simulink model "Filter_Sim_8th_Order"  (R2017a)
settings: Solver=VariableStepAuto  StartTime=0.0  StopTime=t_stop  RelTol=1e-3
values from neighbouring files (symbols this model uses):
  alpha = den_ts    [Filter_Sim.m]
  b_frac = qs    [Filter_Sim.m]
  beta = num_ts    [Filter_Sim.m]
  bw = bi + qs + 1    [Filter_Sim.m]
  bw_accum = 1 + ceil(abs(log2(ts))) + b_frac(2:end)    [Filter_Sim.m]
  k = zeros(1,length(f_norm))    [dIIR_scaling.m]
  shift = round(abs(log2(ts*k)))    [Filter_Sim.m]
  ts = 1/fs    (= 8.85770975057e-08)    [Filter_Sim.m]
libraries: xbsIndex_r4 x117
settings Model: Creator=jpoverelli  LastModifiedBy=jpoverelli

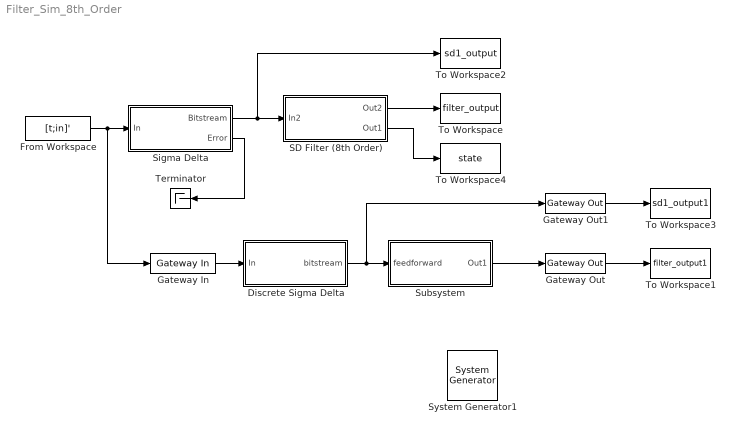
== system Filter_Sim_8th_Order ==
  " System Generator1" : xbsIndex_r4/ System Generator  Tag=genX  xilinxfamily=spartan7  part=xc7s50  speed=-2  package=ftgb196  synthesis_tool=Vivado  clock_wrapper=Clock Enables  directory=/home/jpoverelli/Desktop/Sigma_Delta_Filter_Design/Matlab_Files/Filter_Design/netlist  proj_type=Vivado  Synth_file=Vivado Synthesis Defaults  Impl_file=Vivado Implementation Defaults  testbench=off  simulink_period=ts  sysclk_period=ts/1e-9  dcm_input_clock_period=10  incr_netlist=off  trim_vbits=Everywhere in SubSystem  dbl_ovrd=According to Block Masks  core_generation=According to Block Masks  run_coregen=off  deprecated_control=off  eval_field=0  block_type=sysgen
  Discrete Sigma Delta : Subsystem  mask{bw=bw(1), frac=b_frac(1)}
  From Workspace : FromWorkspace  VariableName=[t;in]'  SampleTime=ts
  Gateway In : xbsIndex_r4/Gateway In  gui_display_data_type=Fixed-point  arith_type="Signed  (2's comp)"  n_bits=bw(1)  bin_pt=b_frac(1)  preci_type=Single  exp_width=8  frac_width=24  rows=1  columns=1  quantization="Round  (unbiased: +/- Inf)"  overflow=Saturate  period=ts  UseAsADC=off  ADCChannel='1'  interface=None  automatic_assignment=on  address_offset=hex2dec('00')  intf_name=''  intf_description=''  default_value=0  timing_constraint=None  locs_specified=off  LOCs={}  io_standard={}  inherit_from_input=off  hdl_port=on  dbl_ovrd=off  block_type=gatewayin
  Gateway Out : xbsIndex_r4/Gateway Out  inherit_from_input=off  hdl_port=on  rows=1  columns=1  UseAsDAC=off  DACChannel='1'  interface=None  automatic_assignment=on  address_offset=hex2dec('00')  intf_name=''  intf_description=''  timing_constraint=None  locs_specified=off  LOCs={}  io_standard={}  block_type=gatewayout
  Gateway Out1 : xbsIndex_r4/Gateway Out  inherit_from_input=off  hdl_port=on  rows=1  columns=1  UseAsDAC=off  DACChannel='1'  interface=None  automatic_assignment=on  address_offset=hex2dec('00')  intf_name=''  intf_description=''  timing_constraint=None  locs_specified=off  LOCs={}  io_standard={}  block_type=gatewayout
  SD Filter (8th Order) : Subsystem
  Sigma Delta : Subsystem
  Subsystem : Subsystem
  Terminator : Terminator
  To Workspace : ToWorkspace  VariableName=filter_output  SampleTime=-1
  To Workspace1 : ToWorkspace  VariableName=filter_output1  SampleTime=-1
  To Workspace2 : ToWorkspace  VariableName=sd1_output  SampleTime=-1
  To Workspace3 : ToWorkspace  VariableName=sd1_output1  SampleTime=-1
  To Workspace4 : ToWorkspace  VariableName=state  SampleTime=-1
  wires:
  From Workspace/1 -> Gateway In/1, Sigma Delta/1(In)
  Sigma Delta/2(Error) -> Terminator/1
  Sigma Delta/1(Bitstream) -> To Workspace2/1, SD Filter (8th Order)/1(In2)
  SD Filter (8th Order)/1(Out2) -> To Workspace/1
  Gateway Out/1 -> To Workspace1/1
  Gateway In/1 -> Discrete Sigma Delta/1(In)
  Subsystem/1(Out1) -> Gateway Out/1
  SD Filter (8th Order)/2(Out1) -> To Workspace4/1
  Discrete Sigma Delta/1(bitstream) -> Gateway Out1/1, Subsystem/1(feedforward)
  Gateway Out1/1 -> To Workspace3/1

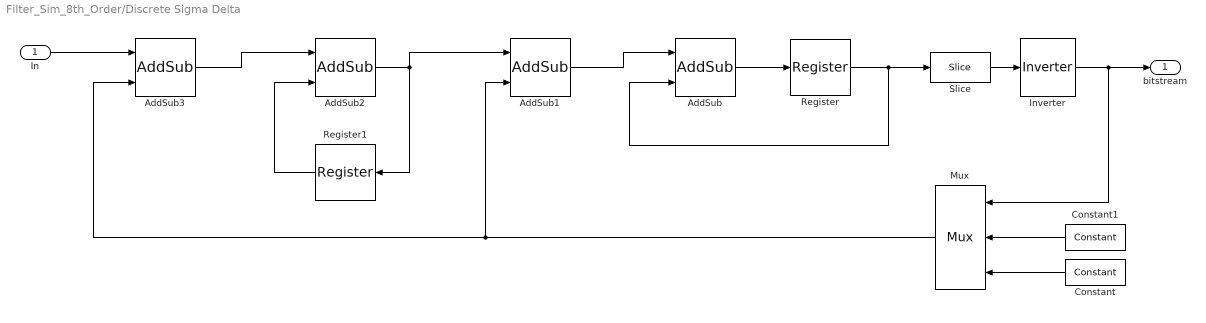
== system Filter_Sim_8th_Order/Discrete Sigma Delta ==
  In : Inport
  AddSub : xbsIndex_r4/AddSub  mode=Addition  use_carryin=off  use_carryout=off  en=off  latency=0  precision=User Defined  arith_type="Signed  (2's comp)"  n_bits=bw+2  bin_pt=frac  quantization="Round  (unbiased: +/- Inf)"  overflow=Saturate  use_behavioral_HDL=off  hw_selection=Fabric  pipelined=off  dbl_ovrd=off  block_type=addsub
  AddSub1 : xbsIndex_r4/AddSub  mode=Subtraction  use_carryin=off  use_carryout=off  en=off  latency=0  precision=User Defined  arith_type="Signed  (2's comp)"  n_bits=bw+2  bin_pt=frac  quantization="Round  (unbiased: +/- Inf)"  overflow=Saturate  use_behavioral_HDL=off  hw_selection=Fabric  pipelined=off  dbl_ovrd=off  block_type=addsub
  AddSub2 : xbsIndex_r4/AddSub  mode=Addition  use_carryin=off  use_carryout=off  en=off  latency=0  precision=User Defined  arith_type="Signed  (2's comp)"  n_bits=bw+2  bin_pt=frac  quantization="Round  (unbiased: +/- Inf)"  overflow=Saturate  use_behavioral_HDL=off  hw_selection=Fabric  pipelined=off  dbl_ovrd=off  block_type=addsub
  AddSub3 : xbsIndex_r4/AddSub  mode=Subtraction  use_carryin=off  use_carryout=off  en=off  latency=0  precision=User Defined  arith_type="Signed  (2's comp)"  n_bits=bw+1  bin_pt=frac  quantization="Round  (unbiased: +/- Inf)"  overflow=Saturate  use_behavioral_HDL=off  hw_selection=Fabric  pipelined=off  dbl_ovrd=off  block_type=addsub
  Constant : xbsIndex_r4/Constant  const=1.0  gui_display_data_type=Fixed-point  arith_type=Signed (2's comp)  n_bits=bw  bin_pt=frac  preci_type=Single  exp_width=8  frac_width=24  explicit_period=off  period=1  equ=P=C  opselect=C  inp2=PCIN>>17  opr=+  inp1=P  carry=CIN  dbl_ovrd=off  block_type=constant
  Constant1 : xbsIndex_r4/Constant  const=-1.0  gui_display_data_type=Fixed-point  arith_type=Signed (2's comp)  n_bits=bw  bin_pt=frac  preci_type=Single  exp_width=8  frac_width=24  explicit_period=off  period=1  equ=P=C  opselect=C  inp2=PCIN>>17  opr=+  inp1=P  carry=CIN  dbl_ovrd=off  block_type=constant
  Inverter : xbsIndex_r4/Inverter  en=off  latency=0  dbl_ovrd=off  block_type=inv
  Mux : xbsIndex_r4/Mux  inputs=2  en=off  latency=0  precision=User Defined  arith_type="Signed  (2's comp)"  n_bits=bw  bin_pt=frac  quantization="Round  (unbiased: +/- Inf)"  overflow=Saturate  dbl_ovrd=off  block_type=mux
  Register : xbsIndex_r4/Register  init=0  rst=off  en=off  dbl_ovrd=off  block_type=register
  Register1 : xbsIndex_r4/Register  init=0  rst=off  en=off  dbl_ovrd=off  block_type=register
  Slice : xbsIndex_r4/Slice  nbits=1  boolean_output=off  mode=Upper Bit Location + Width  bit1=0  base1=MSB of Input  bit0=0  base0=MSB of Input  dbl_ovrd=off  block_type=slice
  bitstream : Outport
  wires:
  AddSub1/1 -> AddSub/1
  Mux/1 -> AddSub3/2, AddSub1/2
  Inverter/1 -> Mux/1, bitstream/1
  Constant/1 -> Mux/3
  AddSub2/1 -> Register1/1, AddSub1/1
  Register1/1 -> AddSub2/2
  Constant1/1 -> Mux/2
  In/1 -> AddSub3/1
  Register/1 -> AddSub/2, Slice/1
  AddSub3/1 -> AddSub2/1
  AddSub/1 -> Register/1
  Slice/1 -> Inverter/1

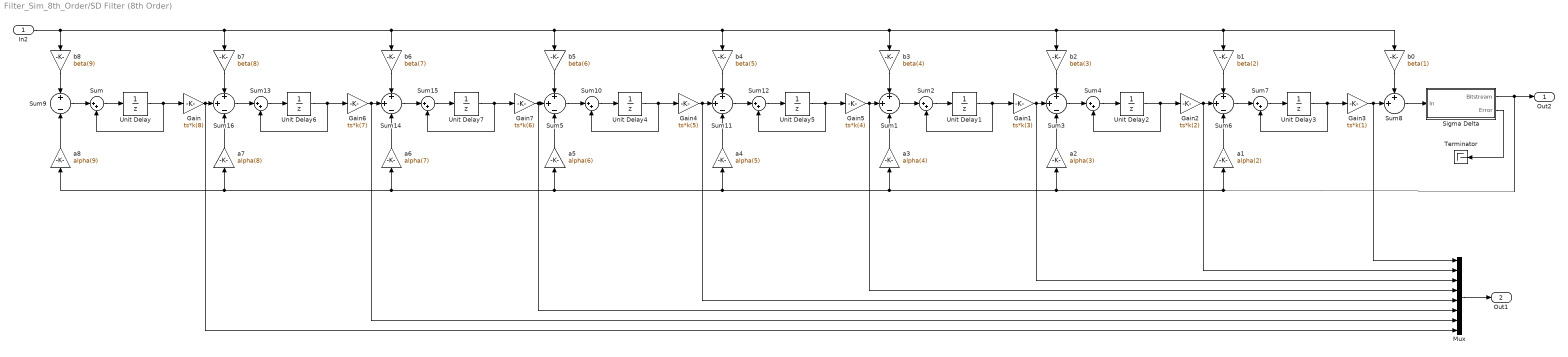
== system Filter_Sim_8th_Order/SD Filter (8th Order) ==
  In2 : Inport
  Gain : Gain  Gain=ts*k(8)  RndMeth=Round
  Gain1 : Gain  Gain=ts*k(3)  RndMeth=Round
  Gain2 : Gain  Gain=ts*k(2)  RndMeth=Round
  Gain3 : Gain  Gain=ts*k(1)  RndMeth=Round
  Gain4 : Gain  Gain=ts*k(5)  RndMeth=Round
  Gain5 : Gain  Gain=ts*k(4)  RndMeth=Round
  Gain6 : Gain  Gain=ts*k(7)  RndMeth=Round
  Gain7 : Gain  Gain=ts*k(6)  RndMeth=Round
  Mux : Mux  Inputs=8
  Sigma Delta : Subsystem
  Sum{,2,4,7,10,12..13,15} (8 alike) : Sum  Inputs=|++
  Sum{1,3,5..6,11,14,16} (7 alike) : Sum  Inputs=+|+|-
  Sum8 : Sum  Inputs=++|
  Sum9 : Sum  Inputs=+|-
  Terminator : Terminator
  Unit Delay{,1..7} (8 alike) : UnitDelay  SampleTime=-1
  a1 : Gain  Gain=alpha(2)
  a2 : Gain  Gain=alpha(3)
  a3 : Gain  Gain=alpha(4)
  a4 : Gain  Gain=alpha(5)
  a5 : Gain  Gain=alpha(6)
  a6 : Gain  Gain=alpha(7)
  a7 : Gain  Gain=alpha(8)
  a8 : Gain  Gain=alpha(9)
  b0 : Gain  Gain=beta(1)
  b1 : Gain  Gain=beta(2)
  b2 : Gain  Gain=beta(3)
  b3 : Gain  Gain=beta(4)
  b4 : Gain  Gain=beta(5)
  b5 : Gain  Gain=beta(6)
  b6 : Gain  Gain=beta(7)
  b7 : Gain  Gain=beta(8)
  b8 : Gain  Gain=beta(9)
  Out2 : Outport
  Out1 : Outport  Port=2
  wires:
  a7/1 -> Sum16/3
  b2/1 -> Sum3/1
  a4/1 -> Sum11/3
  Gain5/1 -> Mux/4, Sum1/2
  Gain7/1 -> Mux/6, Sum5/2
  b3/1 -> Sum1/1
  Sum9/1 -> Sum/1
  Gain2/1 -> Mux/2, Sum6/2
  Sum11/1 -> Sum12/1
  Gain1/1 -> Mux/3, Sum3/2
  Sum10/1 -> Unit Delay4/1
  Sigma Delta/1(Bitstream) -> a1/1, a3/1, a4/1, a5/1, a6/1, a8/1, a7/1, a2/1, Out2/1
  Sum8/1 -> Sigma Delta/1(In)
  Sum7/1 -> Unit Delay3/1
  In2/1 -> b0/1, b1/1, b2/1, b3/1, b4/1, b5/1, b6/1, b7/1, b8/1
  Gain3/1 -> Mux/1, Sum8/2
  Sum4/1 -> Unit Delay2/1
  a3/1 -> Sum1/3
  Unit Delay6/1 -> Sum13/2, Gain6/1
  Sum2/1 -> Unit Delay1/1
  Sum6/1 -> Sum7/1
  Unit Delay3/1 -> Sum7/2, Gain3/1
  Sum/1 -> Unit Delay/1
  Gain6/1 -> Mux/7, Sum14/2
  Sum14/1 -> Sum15/1
  a5/1 -> Sum5/3
  Sum13/1 -> Unit Delay6/1
  b5/1 -> Sum5/1
  Gain4/1 -> Mux/5, Sum11/2
  a2/1 -> Sum3/3
  Unit Delay4/1 -> Sum10/2, Gain4/1
  Sum5/1 -> Sum10/1
  Sigma Delta/2(Error) -> Terminator/1
  b1/1 -> Sum6/1
  Sum1/1 -> Sum2/1
  a1/1 -> Sum6/3
  Sum15/1 -> Unit Delay7/1
  Unit Delay1/1 -> Sum2/2, Gain1/1
  b8/1 -> Sum9/1
  Unit Delay5/1 -> Sum12/2, Gain5/1
  Unit Delay2/1 -> Sum4/2, Gain2/1
  Unit Delay/1 -> Sum/2, Gain/1
  Gain/1 -> Mux/8, Sum16/2
  b6/1 -> Sum14/1
  b4/1 -> Sum11/1
  Unit Delay7/1 -> Sum15/2, Gain7/1
  Sum3/1 -> Sum4/1
  a6/1 -> Sum14/3
  Sum12/1 -> Unit Delay5/1
  Sum16/1 -> Sum13/1
  b7/1 -> Sum16/1
  a8/1 -> Sum9/2
  b0/1 -> Sum8/1
  Mux/1 -> Out1/1

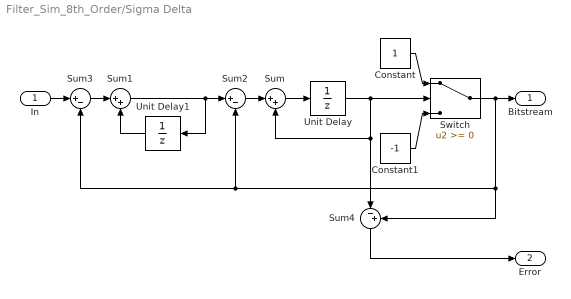
== system Filter_Sim_8th_Order/Sigma Delta ==
  In : Inport
  Constant : Constant
  Constant1 : Constant  Value=-1
  Sum : Sum  Inputs=|++
  Sum1 : Sum  Inputs=|++
  Sum2 : Sum  Inputs=|+-
  Sum3 : Sum  Inputs=|+-
  Sum4 : Sum  Inputs=|-+
  Switch : Switch
  Unit Delay : UnitDelay  SampleTime=ts
  Unit Delay1 : UnitDelay  SampleTime=ts
  Bitstream : Outport
  Error : Outport  Port=2
  wires:
  Sum4/1 -> Error/1
  Sum3/1 -> Sum1/1
  Switch/1 -> Sum4/2, Sum2/2, Sum3/2, Bitstream/1
  Constant1/1 -> Switch/3
  Unit Delay1/1 -> Sum1/2
  Sum/1 -> Unit Delay/1
  Unit Delay/1 -> Sum4/1, Sum/2, Switch/2
  Constant/1 -> Switch/1
  In/1 -> Sum3/1
  Sum2/1 -> Sum/1
  Sum1/1 -> Sum2/1, Unit Delay1/1

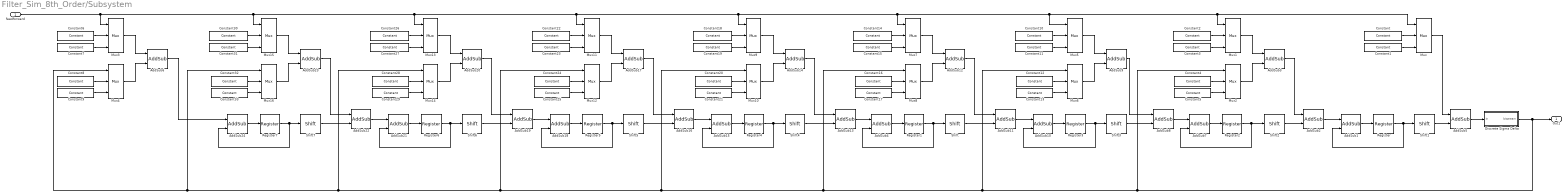
== system Filter_Sim_8th_Order/Subsystem ==
  feedforward : Inport
  AddSub1 : xbsIndex_r4/AddSub  mode=Addition  use_carryin=off  use_carryout=off  en=off  latency=0  precision=User Defined  arith_type="Signed  (2's comp)"  n_bits=bw_accum(1)  bin_pt=b_frac(2)  quantization="Round  (unbiased: +/- Inf)"  overflow=Saturate  use_behavioral_HDL=off  hw_selection=Fabric  pipelined=off  dbl_ovrd=off  block_type=addsub
  AddSub10 : xbsIndex_r4/AddSub  mode=Addition  use_carryin=off  use_carryout=off  en=off  latency=0  precision=User Defined  arith_type="Signed  (2's comp)"  n_bits=bw_accum(3)  bin_pt=b_frac(4)  quantization="Round  (unbiased: +/- Inf)"  overflow=Saturate  use_behavioral_HDL=off  hw_selection=Fabric  pipelined=off  dbl_ovrd=off  block_type=addsub
  AddSub11 : xbsIndex_r4/AddSub  mode=Addition  use_carryin=off  use_carryout=off  en=off  latency=0  precision=User Defined  arith_type="Signed  (2's comp)"  n_bits=bw_accum(3)  bin_pt=b_frac(4)  quantization="Round  (unbiased: +/- Inf)"  overflow=Saturate  use_behavioral_HDL=off  hw_selection=Fabric  pipelined=off  dbl_ovrd=off  block_type=addsub
  AddSub12 : xbsIndex_r4/AddSub  mode=Subtraction  use_carryin=off  use_carryout=off  en=off  latency=0  precision=User Defined  arith_type="Signed  (2's comp)"  n_bits=bw(4)  bin_pt=b_frac(4)  quantization="Round  (unbiased: +/- Inf)"  overflow=Saturate  use_behavioral_HDL=off  hw_selection=Fabric  pipelined=off  dbl_ovrd=off  block_type=addsub
  AddSub13 : xbsIndex_r4/AddSub  mode=Addition  use_carryin=off  use_carryout=off  en=off  latency=0  precision=User Defined  arith_type="Signed  (2's comp)"  n_bits=bw_accum(4)  bin_pt=b_frac(5)  quantization="Round  (unbiased: +/- Inf)"  overflow=Saturate  use_behavioral_HDL=off  hw_selection=Fabric  pipelined=off  dbl_ovrd=off  block_type=addsub
  AddSub14 : xbsIndex_r4/AddSub  mode=Subtraction  use_carryin=off  use_carryout=off  en=off  latency=0  precision=User Defined  arith_type="Signed  (2's comp)"  n_bits=bw(5)  bin_pt=b_frac(5)  quantization="Round  (unbiased: +/- Inf)"  overflow=Saturate  use_behavioral_HDL=off  hw_selection=Fabric  pipelined=off  dbl_ovrd=off  block_type=addsub
  AddSub15 : xbsIndex_r4/AddSub  mode=Addition  use_carryin=off  use_carryout=off  en=off  latency=0  precision=User Defined  arith_type="Signed  (2's comp)"  n_bits=bw_accum(5)  bin_pt=b_frac(6)  quantization="Round  (unbiased: +/- Inf)"  overflow=Saturate  use_behavioral_HDL=off  hw_selection=Fabric  pipelined=off  dbl_ovrd=off  block_type=addsub
  AddSub16 : xbsIndex_r4/AddSub  mode=Addition  use_carryin=off  use_carryout=off  en=off  latency=0  precision=User Defined  arith_type="Signed  (2's comp)"  n_bits=bw_accum(5)  bin_pt=b_frac(6)  quantization="Round  (unbiased: +/- Inf)"  overflow=Saturate  use_behavioral_HDL=off  hw_selection=Fabric  pipelined=off  dbl_ovrd=off  block_type=addsub
  AddSub17 : xbsIndex_r4/AddSub  mode=Subtraction  use_carryin=off  use_carryout=off  en=off  latency=0  precision=User Defined  arith_type="Signed  (2's comp)"  n_bits=bw(6)  bin_pt=b_frac(6)  quantization="Round  (unbiased: +/- Inf)"  overflow=Saturate  use_behavioral_HDL=off  hw_selection=Fabric  pipelined=off  dbl_ovrd=off  block_type=addsub
  AddSub18 : xbsIndex_r4/AddSub  mode=Addition  use_carryin=off  use_carryout=off  en=off  latency=0  precision=User Defined  arith_type="Signed  (2's comp)"  n_bits=bw_accum(6)  bin_pt=b_frac(7)  quantization="Round  (unbiased: +/- Inf)"  overflow=Saturate  use_behavioral_HDL=off  hw_selection=Fabric  pipelined=off  dbl_ovrd=off  block_type=addsub
  AddSub19 : xbsIndex_r4/AddSub  mode=Addition  use_carryin=off  use_carryout=off  en=off  latency=0  precision=User Defined  arith_type="Signed  (2's comp)"  n_bits=bw_accum(6)  bin_pt=b_frac(7)  quantization="Round  (unbiased: +/- Inf)"  overflow=Saturate  use_behavioral_HDL=off  hw_selection=Fabric  pipelined=off  dbl_ovrd=off  block_type=addsub
  AddSub2 : xbsIndex_r4/AddSub  mode=Addition  use_carryin=off  use_carryout=off  en=off  latency=0  precision=User Defined  arith_type="Signed  (2's comp)"  n_bits=bw_accum(1)  bin_pt=b_frac(2)  quantization="Round  (unbiased: +/- Inf)"  overflow=Saturate  use_behavioral_HDL=off  hw_selection=Fabric  pipelined=off  dbl_ovrd=off  block_type=addsub
  AddSub20 : xbsIndex_r4/AddSub  mode=Subtraction  use_carryin=off  use_carryout=off  en=off  latency=0  precision=User Defined  arith_type="Signed  (2's comp)"  n_bits=bw(7)  bin_pt=b_frac(7)  quantization="Round  (unbiased: +/- Inf)"  overflow=Saturate  use_behavioral_HDL=off  hw_selection=Fabric  pipelined=off  dbl_ovrd=off  block_type=addsub
  AddSub21 : xbsIndex_r4/AddSub  mode=Addition  use_carryin=off  use_carryout=off  en=off  latency=0  precision=User Defined  arith_type="Signed  (2's comp)"  n_bits=bw_accum(7)  bin_pt=b_frac(8)  quantization="Round  (unbiased: +/- Inf)"  overflow=Saturate  use_behavioral_HDL=off  hw_selection=Fabric  pipelined=off  dbl_ovrd=off  block_type=addsub
  AddSub22 : xbsIndex_r4/AddSub  mode=Addition  use_carryin=off  use_carryout=off  en=off  latency=0  precision=User Defined  arith_type="Signed  (2's comp)"  n_bits=bw_accum(7)  bin_pt=b_frac(8)  quantization="Round  (unbiased: +/- Inf)"  overflow=Saturate  use_behavioral_HDL=off  hw_selection=Fabric  pipelined=off  dbl_ovrd=off  block_type=addsub
  AddSub23 : xbsIndex_r4/AddSub  mode=Subtraction  use_carryin=off  use_carryout=off  en=off  latency=0  precision=User Defined  arith_type="Signed  (2's comp)"  n_bits=bw(8)  bin_pt=b_frac(8)  quantization="Round  (unbiased: +/- Inf)"  overflow=Saturate  use_behavioral_HDL=off  hw_selection=Fabric  pipelined=off  dbl_ovrd=off  block_type=addsub
  AddSub24 : xbsIndex_r4/AddSub  mode=Addition  use_carryin=off  use_carryout=off  en=off  latency=0  precision=User Defined  arith_type="Signed  (2's comp)"  n_bits=bw_accum(8)  bin_pt=b_frac(9)  quantization="Round  (unbiased: +/- Inf)"  overflow=Saturate  use_behavioral_HDL=off  hw_selection=Fabric  pipelined=off  dbl_ovrd=off  block_type=addsub
  AddSub3 : xbsIndex_r4/AddSub  mode=Subtraction  use_carryin=off  use_carryout=off  en=off  latency=0  precision=User Defined  arith_type="Signed  (2's comp)"  n_bits=bw(2)  bin_pt=b_frac(2)  quantization="Round  (unbiased: +/- Inf)"  overflow=Saturate  use_behavioral_HDL=off  hw_selection=Fabric  pipelined=off  dbl_ovrd=off  block_type=addsub
  AddSub4 : xbsIndex_r4/AddSub  mode=Addition  use_carryin=off  use_carryout=off  en=off  latency=0  precision=User Defined  arith_type="Signed  (2's comp)"  n_bits=bw_accum(4)  bin_pt=b_frac(5)  quantization="Round  (unbiased: +/- Inf)"  overflow=Saturate  use_behavioral_HDL=off  hw_selection=Fabric  pipelined=off  dbl_ovrd=off  block_type=addsub
  AddSub5 : xbsIndex_r4/AddSub  mode=Addition  use_carryin=off  use_carryout=off  en=off  latency=0  precision=User Defined  arith_type="Signed  (2's comp)"  n_bits=bw(1)  bin_pt=b_frac(1)  quantization="Round  (unbiased: +/- Inf)"  overflow=Saturate  use_behavioral_HDL=off  hw_selection=Fabric  pipelined=off  dbl_ovrd=off  block_type=addsub
  AddSub6 : xbsIndex_r4/AddSub  mode=Subtraction  use_carryin=off  use_carryout=off  en=off  latency=0  precision=User Defined  arith_type="Signed  (2's comp)"  n_bits=bw(9)  bin_pt=b_frac(9)  quantization="Round  (unbiased: +/- Inf)"  overflow=Saturate  use_behavioral_HDL=off  hw_selection=Fabric  pipelined=off  dbl_ovrd=off  block_type=addsub
  AddSub7 : xbsIndex_r4/AddSub  mode=Addition  use_carryin=off  use_carryout=off  en=off  latency=0  precision=User Defined  arith_type="Signed  (2's comp)"  n_bits=bw_accum(2)  bin_pt=b_frac(3)  quantization="Round  (unbiased: +/- Inf)"  overflow=Saturate  use_behavioral_HDL=off  hw_selection=Fabric  pipelined=off  dbl_ovrd=off  block_type=addsub
  AddSub8 : xbsIndex_r4/AddSub  mode=Addition  use_carryin=off  use_carryout=off  en=off  latency=0  precision=User Defined  arith_type="Signed  (2's comp)"  n_bits=bw_accum(2)  bin_pt=b_frac(3)  quantization="Round  (unbiased: +/- Inf)"  overflow=Saturate  use_behavioral_HDL=off  hw_selection=Fabric  pipelined=off  dbl_ovrd=off  block_type=addsub
  AddSub9 : xbsIndex_r4/AddSub  mode=Subtraction  use_carryin=off  use_carryout=off  en=off  latency=0  precision=User Defined  arith_type="Signed  (2's comp)"  n_bits=bw(3)  bin_pt=b_frac(3)  quantization="Round  (unbiased: +/- Inf)"  overflow=Saturate  use_behavioral_HDL=off  hw_selection=Fabric  pipelined=off  dbl_ovrd=off  block_type=addsub
  Constant : xbsIndex_r4/Constant  const=-beta(1)  gui_display_data_type=Fixed-point  arith_type=Signed (2's comp)  n_bits=bw(1)  bin_pt=b_frac(1)  preci_type=Single  exp_width=8  frac_width=24  explicit_period=off  period=1  equ=P=C  opselect=C  inp2=PCIN>>17  opr=+  inp1=P  carry=CIN  dbl_ovrd=off  block_type=constant
  Constant1 : xbsIndex_r4/Constant  const=beta(1)  gui_display_data_type=Fixed-point  arith_type=Signed (2's comp)  n_bits=bw(1)  bin_pt=b_frac(1)  preci_type=Single  exp_width=8  frac_width=24  explicit_period=off  period=1  equ=P=C  opselect=C  inp2=PCIN>>17  opr=+  inp1=P  carry=CIN  dbl_ovrd=off  block_type=constant
  Constant10 : xbsIndex_r4/Constant  const=-beta(3)  gui_display_data_type=Fixed-point  arith_type=Signed (2's comp)  n_bits=bw(3)  bin_pt=b_frac(3)  preci_type=Single  exp_width=8  frac_width=24  explicit_period=off  period=1  equ=P=C  opselect=C  inp2=PCIN>>17  opr=+  inp1=P  carry=CIN  dbl_ovrd=off  block_type=constant
  Constant11 : xbsIndex_r4/Constant  const=beta(3)  gui_display_data_type=Fixed-point  arith_type=Signed (2's comp)  n_bits=bw(3)  bin_pt=b_frac(3)  preci_type=Single  exp_width=8  frac_width=24  explicit_period=off  period=1  equ=P=C  opselect=C  inp2=PCIN>>17  opr=+  inp1=P  carry=CIN  dbl_ovrd=off  block_type=constant
  Constant12 : xbsIndex_r4/Constant  const=-alpha(3)  gui_display_data_type=Fixed-point  arith_type=Signed (2's comp)  n_bits=bw(3)  bin_pt=b_frac(3)  preci_type=Single  exp_width=8  frac_width=24  explicit_period=off  period=1  equ=P=C  opselect=C  inp2=PCIN>>17  opr=+  inp1=P  carry=CIN  dbl_ovrd=off  block_type=constant
  Constant13 : xbsIndex_r4/Constant  const=alpha(3)  gui_display_data_type=Fixed-point  arith_type=Signed (2's comp)  n_bits=bw(3)  bin_pt=b_frac(3)  preci_type=Single  exp_width=8  frac_width=24  explicit_period=off  period=1  equ=P=C  opselect=C  inp2=PCIN>>17  opr=+  inp1=P  carry=CIN  dbl_ovrd=off  block_type=constant
  Constant14 : xbsIndex_r4/Constant  const=-beta(4)  gui_display_data_type=Fixed-point  arith_type=Signed (2's comp)  n_bits=bw(4)  bin_pt=b_frac(4)  preci_type=Single  exp_width=8  frac_width=24  explicit_period=off  period=1  equ=P=C  opselect=C  inp2=PCIN>>17  opr=+  inp1=P  carry=CIN  dbl_ovrd=off  block_type=constant
  Constant15 : xbsIndex_r4/Constant  const=beta(4)  gui_display_data_type=Fixed-point  arith_type=Signed (2's comp)  n_bits=bw(4)  bin_pt=b_frac(4)  preci_type=Single  exp_width=8  frac_width=24  explicit_period=off  period=1  equ=P=C  opselect=C  inp2=PCIN>>17  opr=+  inp1=P  carry=CIN  dbl_ovrd=off  block_type=constant
  Constant16 : xbsIndex_r4/Constant  const=-alpha(4)  gui_display_data_type=Fixed-point  arith_type=Signed (2's comp)  n_bits=bw(4)  bin_pt=b_frac(4)  preci_type=Single  exp_width=8  frac_width=24  explicit_period=off  period=1  equ=P=C  opselect=C  inp2=PCIN>>17  opr=+  inp1=P  carry=CIN  dbl_ovrd=off  block_type=constant
  Constant17 : xbsIndex_r4/Constant  const=alpha(4)  gui_display_data_type=Fixed-point  arith_type=Signed (2's comp)  n_bits=bw(4)  bin_pt=b_frac(4)  preci_type=Single  exp_width=8  frac_width=24  explicit_period=off  period=1  equ=P=C  opselect=C  inp2=PCIN>>17  opr=+  inp1=P  carry=CIN  dbl_ovrd=off  block_type=constant
  Constant18 : xbsIndex_r4/Constant  const=-beta(5)  gui_display_data_type=Fixed-point  arith_type=Signed (2's comp)  n_bits=bw(5)  bin_pt=b_frac(5)  preci_type=Single  exp_width=8  frac_width=24  explicit_period=off  period=1  equ=P=C  opselect=C  inp2=PCIN>>17  opr=+  inp1=P  carry=CIN  dbl_ovrd=off  block_type=constant
  Constant19 : xbsIndex_r4/Constant  const=beta(5)  gui_display_data_type=Fixed-point  arith_type=Signed (2's comp)  n_bits=bw(5)  bin_pt=b_frac(5)  preci_type=Single  exp_width=8  frac_width=24  explicit_period=off  period=1  equ=P=C  opselect=C  inp2=PCIN>>17  opr=+  inp1=P  carry=CIN  dbl_ovrd=off  block_type=constant
  Constant2 : xbsIndex_r4/Constant  const=-beta(2)  gui_display_data_type=Fixed-point  arith_type=Signed (2's comp)  n_bits=bw(2)  bin_pt=b_frac(2)  preci_type=Single  exp_width=8  frac_width=24  explicit_period=off  period=1  equ=P=C  opselect=C  inp2=PCIN>>17  opr=+  inp1=P  carry=CIN  dbl_ovrd=off  block_type=constant
  Constant20 : xbsIndex_r4/Constant  const=-alpha(5)  gui_display_data_type=Fixed-point  arith_type=Signed (2's comp)  n_bits=bw(5)  bin_pt=b_frac(5)  preci_type=Single  exp_width=8  frac_width=24  explicit_period=off  period=1  equ=P=C  opselect=C  inp2=PCIN>>17  opr=+  inp1=P  carry=CIN  dbl_ovrd=off  block_type=constant
  Constant21 : xbsIndex_r4/Constant  const=alpha(5)  gui_display_data_type=Fixed-point  arith_type=Signed (2's comp)  n_bits=bw(5)  bin_pt=b_frac(5)  preci_type=Single  exp_width=8  frac_width=24  explicit_period=off  period=1  equ=P=C  opselect=C  inp2=PCIN>>17  opr=+  inp1=P  carry=CIN  dbl_ovrd=off  block_type=constant
  Constant22 : xbsIndex_r4/Constant  const=-beta(6)  gui_display_data_type=Fixed-point  arith_type=Signed (2's comp)  n_bits=bw(6)  bin_pt=b_frac(6)  preci_type=Single  exp_width=8  frac_width=24  explicit_period=off  period=1  equ=P=C  opselect=C  inp2=PCIN>>17  opr=+  inp1=P  carry=CIN  dbl_ovrd=off  block_type=constant
  Constant23 : xbsIndex_r4/Constant  const=beta(6)  gui_display_data_type=Fixed-point  arith_type=Signed (2's comp)  n_bits=bw(6)  bin_pt=b_frac(6)  preci_type=Single  exp_width=8  frac_width=24  explicit_period=off  period=1  equ=P=C  opselect=C  inp2=PCIN>>17  opr=+  inp1=P  carry=CIN  dbl_ovrd=off  block_type=constant
  Constant24 : xbsIndex_r4/Constant  const=-alpha(6)  gui_display_data_type=Fixed-point  arith_type=Signed (2's comp)  n_bits=bw(6)  bin_pt=b_frac(6)  preci_type=Single  exp_width=8  frac_width=24  explicit_period=off  period=1  equ=P=C  opselect=C  inp2=PCIN>>17  opr=+  inp1=P  carry=CIN  dbl_ovrd=off  block_type=constant
  Constant25 : xbsIndex_r4/Constant  const=alpha(6)  gui_display_data_type=Fixed-point  arith_type=Signed (2's comp)  n_bits=bw(6)  bin_pt=b_frac(6)  preci_type=Single  exp_width=8  frac_width=24  explicit_period=off  period=1  equ=P=C  opselect=C  inp2=PCIN>>17  opr=+  inp1=P  carry=CIN  dbl_ovrd=off  block_type=constant
  Constant26 : xbsIndex_r4/Constant  const=-beta(7)  gui_display_data_type=Fixed-point  arith_type=Signed (2's comp)  n_bits=bw(7)  bin_pt=b_frac(7)  preci_type=Single  exp_width=8  frac_width=24  explicit_period=off  period=1  equ=P=C  opselect=C  inp2=PCIN>>17  opr=+  inp1=P  carry=CIN  dbl_ovrd=off  block_type=constant
  Constant27 : xbsIndex_r4/Constant  const=beta(7)  gui_display_data_type=Fixed-point  arith_type=Signed (2's comp)  n_bits=bw(7)  bin_pt=b_frac(7)  preci_type=Single  exp_width=8  frac_width=24  explicit_period=off  period=1  equ=P=C  opselect=C  inp2=PCIN>>17  opr=+  inp1=P  carry=CIN  dbl_ovrd=off  block_type=constant
  Constant28 : xbsIndex_r4/Constant  const=-alpha(7)  gui_display_data_type=Fixed-point  arith_type=Signed (2's comp)  n_bits=bw(7)  bin_pt=b_frac(7)  preci_type=Single  exp_width=8  frac_width=24  explicit_period=off  period=1  equ=P=C  opselect=C  inp2=PCIN>>17  opr=+  inp1=P  carry=CIN  dbl_ovrd=off  block_type=constant
  Constant29 : xbsIndex_r4/Constant  const=alpha(7)  gui_display_data_type=Fixed-point  arith_type=Signed (2's comp)  n_bits=bw(7)  bin_pt=b_frac(7)  preci_type=Single  exp_width=8  frac_width=24  explicit_period=off  period=1  equ=P=C  opselect=C  inp2=PCIN>>17  opr=+  inp1=P  carry=CIN  dbl_ovrd=off  block_type=constant
  Constant3 : xbsIndex_r4/Constant  const=beta(2)  gui_display_data_type=Fixed-point  arith_type=Signed (2's comp)  n_bits=bw(2)  bin_pt=b_frac(2)  preci_type=Single  exp_width=8  frac_width=24  explicit_period=off  period=1  equ=P=C  opselect=C  inp2=PCIN>>17  opr=+  inp1=P  carry=CIN  dbl_ovrd=off  block_type=constant
  Constant30 : xbsIndex_r4/Constant  const=-beta(8)  gui_display_data_type=Fixed-point  arith_type=Signed (2's comp)  n_bits=bw(8)  bin_pt=b_frac(8)  preci_type=Single  exp_width=8  frac_width=24  explicit_period=off  period=1  equ=P=C  opselect=C  inp2=PCIN>>17  opr=+  inp1=P  carry=CIN  dbl_ovrd=off  block_type=constant
  Constant31 : xbsIndex_r4/Constant  const=beta(8)  gui_display_data_type=Fixed-point  arith_type=Signed (2's comp)  n_bits=bw(8)  bin_pt=b_frac(8)  preci_type=Single  exp_width=8  frac_width=24  explicit_period=off  period=1  equ=P=C  opselect=C  inp2=PCIN>>17  opr=+  inp1=P  carry=CIN  dbl_ovrd=off  block_type=constant
  Constant32 : xbsIndex_r4/Constant  const=-alpha(8)  gui_display_data_type=Fixed-point  arith_type=Signed (2's comp)  n_bits=bw(8)  bin_pt=b_frac(8)  preci_type=Single  exp_width=8  frac_width=24  explicit_period=off  period=1  equ=P=C  opselect=C  inp2=PCIN>>17  opr=+  inp1=P  carry=CIN  dbl_ovrd=off  block_type=constant
  Constant33 : xbsIndex_r4/Constant  const=alpha(8)  gui_display_data_type=Fixed-point  arith_type=Signed (2's comp)  n_bits=bw(8)  bin_pt=b_frac(8)  preci_type=Single  exp_width=8  frac_width=24  explicit_period=off  period=1  equ=P=C  opselect=C  inp2=PCIN>>17  opr=+  inp1=P  carry=CIN  dbl_ovrd=off  block_type=constant
  Constant4 : xbsIndex_r4/Constant  const=-alpha(2)  gui_display_data_type=Fixed-point  arith_type=Signed (2's comp)  n_bits=bw(2)  bin_pt=b_frac(2)  preci_type=Single  exp_width=8  frac_width=24  explicit_period=off  period=1  equ=P=C  opselect=C  inp2=PCIN>>17  opr=+  inp1=P  carry=CIN  dbl_ovrd=off  block_type=constant
  Constant5 : xbsIndex_r4/Constant  const=alpha(2)  gui_display_data_type=Fixed-point  arith_type=Signed (2's comp)  n_bits=bw(2)  bin_pt=b_frac(2)  preci_type=Single  exp_width=8  frac_width=24  explicit_period=off  period=1  equ=P=C  opselect=C  inp2=PCIN>>17  opr=+  inp1=P  carry=CIN  dbl_ovrd=off  block_type=constant
  Constant6 : xbsIndex_r4/Constant  const=-beta(9)  gui_display_data_type=Fixed-point  arith_type=Signed (2's comp)  n_bits=bw(9)  bin_pt=b_frac(9)  preci_type=Single  exp_width=8  frac_width=24  explicit_period=off  period=1  equ=P=C  opselect=C  inp2=PCIN>>17  opr=+  inp1=P  carry=CIN  dbl_ovrd=off  block_type=constant
  Constant7 : xbsIndex_r4/Constant  const=beta(9)  gui_display_data_type=Fixed-point  arith_type=Signed (2's comp)  n_bits=bw(9)  bin_pt=b_frac(9)  preci_type=Single  exp_width=8  frac_width=24  explicit_period=off  period=1  equ=P=C  opselect=C  inp2=PCIN>>17  opr=+  inp1=P  carry=CIN  dbl_ovrd=off  block_type=constant
  Constant8 : xbsIndex_r4/Constant  const=-alpha(9)  gui_display_data_type=Fixed-point  arith_type=Signed (2's comp)  n_bits=bw(9)  bin_pt=b_frac(9)  preci_type=Single  exp_width=8  frac_width=24  explicit_period=off  period=1  equ=P=C  opselect=C  inp2=PCIN>>17  opr=+  inp1=P  carry=CIN  dbl_ovrd=off  block_type=constant
  Constant9 : xbsIndex_r4/Constant  const=alpha(9)  gui_display_data_type=Fixed-point  arith_type=Signed (2's comp)  n_bits=bw(9)  bin_pt=b_frac(9)  preci_type=Single  exp_width=8  frac_width=24  explicit_period=off  period=1  equ=P=C  opselect=C  inp2=PCIN>>17  opr=+  inp1=P  carry=CIN  dbl_ovrd=off  block_type=constant
  Discrete Sigma Delta : Subsystem  mask{bw=bw(1), frac=b_frac(1)}
  Mux : xbsIndex_r4/Mux  inputs=2  en=off  latency=0  precision=User Defined  arith_type="Signed  (2's comp)"  n_bits=bw(1)  bin_pt=b_frac(1)  quantization="Round  (unbiased: +/- Inf)"  overflow=Saturate  dbl_ovrd=off  block_type=mux
  Mux1 : xbsIndex_r4/Mux  inputs=2  en=off  latency=0  precision=User Defined  arith_type="Signed  (2's comp)"  n_bits=bw(2)  bin_pt=b_frac(2)  quantization="Round  (unbiased: +/- Inf)"  overflow=Saturate  dbl_ovrd=off  block_type=mux
  Mux10 : xbsIndex_r4/Mux  inputs=2  en=off  latency=0  precision=User Defined  arith_type="Signed  (2's comp)"  n_bits=bw(5)  bin_pt=b_frac(5)  quantization="Round  (unbiased: +/- Inf)"  overflow=Saturate  dbl_ovrd=off  block_type=mux
  Mux11 : xbsIndex_r4/Mux  inputs=2  en=off  latency=0  precision=User Defined  arith_type="Signed  (2's comp)"  n_bits=bw(6)  bin_pt=b_frac(6)  quantization="Round  (unbiased: +/- Inf)"  overflow=Saturate  dbl_ovrd=off  block_type=mux
  Mux12 : xbsIndex_r4/Mux  inputs=2  en=off  latency=0  precision=User Defined  arith_type="Signed  (2's comp)"  n_bits=bw(6)  bin_pt=b_frac(6)  quantization="Round  (unbiased: +/- Inf)"  overflow=Saturate  dbl_ovrd=off  block_type=mux
  Mux13 : xbsIndex_r4/Mux  inputs=2  en=off  latency=0  precision=User Defined  arith_type="Signed  (2's comp)"  n_bits=bw(7)  bin_pt=b_frac(7)  quantization="Round  (unbiased: +/- Inf)"  overflow=Saturate  dbl_ovrd=off  block_type=mux
  Mux14 : xbsIndex_r4/Mux  inputs=2  en=off  latency=0  precision=User Defined  arith_type="Signed  (2's comp)"  n_bits=bw(7)  bin_pt=b_frac(7)  quantization="Round  (unbiased: +/- Inf)"  overflow=Saturate  dbl_ovrd=off  block_type=mux
  Mux15 : xbsIndex_r4/Mux  inputs=2  en=off  latency=0  precision=User Defined  arith_type="Signed  (2's comp)"  n_bits=bw(8)  bin_pt=b_frac(8)  quantization="Round  (unbiased: +/- Inf)"  overflow=Saturate  dbl_ovrd=off  block_type=mux
  Mux16 : xbsIndex_r4/Mux  inputs=2  en=off  latency=0  precision=User Defined  arith_type="Signed  (2's comp)"  n_bits=bw(8)  bin_pt=b_frac(8)  quantization="Round  (unbiased: +/- Inf)"  overflow=Saturate  dbl_ovrd=off  block_type=mux
  Mux2 : xbsIndex_r4/Mux  inputs=2  en=off  latency=0  precision=User Defined  arith_type="Signed  (2's comp)"  n_bits=bw(2)  bin_pt=b_frac(2)  quantization="Round  (unbiased: +/- Inf)"  overflow=Saturate  dbl_ovrd=off  block_type=mux
  Mux3 : xbsIndex_r4/Mux  inputs=2  en=off  latency=0  precision=User Defined  arith_type="Signed  (2's comp)"  n_bits=bw(9)  bin_pt=b_frac(9)  quantization="Round  (unbiased: +/- Inf)"  overflow=Saturate  dbl_ovrd=off  block_type=mux
  Mux4 : xbsIndex_r4/Mux  inputs=2  en=off  latency=0  precision=User Defined  arith_type="Signed  (2's comp)"  n_bits=bw(9)  bin_pt=b_frac(9)  quantization="Round  (unbiased: +/- Inf)"  overflow=Saturate  dbl_ovrd=off  block_type=mux
  Mux5 : xbsIndex_r4/Mux  inputs=2  en=off  latency=0  precision=User Defined  arith_type="Signed  (2's comp)"  n_bits=bw(3)  bin_pt=b_frac(3)  quantization="Round  (unbiased: +/- Inf)"  overflow=Saturate  dbl_ovrd=off  block_type=mux
  Mux6 : xbsIndex_r4/Mux  inputs=2  en=off  latency=0  precision=User Defined  arith_type="Signed  (2's comp)"  n_bits=bw(3)  bin_pt=b_frac(3)  quantization="Round  (unbiased: +/- Inf)"  overflow=Saturate  dbl_ovrd=off  block_type=mux
  Mux7 : xbsIndex_r4/Mux  inputs=2  en=off  latency=0  precision=User Defined  arith_type="Signed  (2's comp)"  n_bits=bw(4)  bin_pt=b_frac(4)  quantization="Round  (unbiased: +/- Inf)"  overflow=Saturate  dbl_ovrd=off  block_type=mux
  Mux8 : xbsIndex_r4/Mux  inputs=2  en=off  latency=0  precision=User Defined  arith_type="Signed  (2's comp)"  n_bits=bw(4)  bin_pt=b_frac(4)  quantization="Round  (unbiased: +/- Inf)"  overflow=Saturate  dbl_ovrd=off  block_type=mux
  Mux9 : xbsIndex_r4/Mux  inputs=2  en=off  latency=0  precision=User Defined  arith_type="Signed  (2's comp)"  n_bits=bw(5)  bin_pt=b_frac(5)  quantization="Round  (unbiased: +/- Inf)"  overflow=Saturate  dbl_ovrd=off  block_type=mux
  Register{,1..7} (8 alike) : xbsIndex_r4/Register  init=0  rst=off  en=off  dbl_ovrd=off  block_type=register
  Shift : xbsIndex_r4/Shift  shift_dir=Right  shift_bits=shift(4)  en=off  latency=0  precision=User Defined  arith_type="Signed  (2's comp)"  n_bits=bw(4)  bin_pt=b_frac(4)  quantization="Round  (unbiased: +/- Inf)"  overflow=Saturate  dbl_ovrd=off  block_type=shift
  Shift1 : xbsIndex_r4/Shift  shift_dir=Right  shift_bits=shift(1)  en=off  latency=0  precision=User Defined  arith_type="Signed  (2's comp)"  n_bits=bw(1)  bin_pt=b_frac(1)  quantization="Round  (unbiased: +/- Inf)"  overflow=Saturate  dbl_ovrd=off  block_type=shift
  Shift2 : xbsIndex_r4/Shift  shift_dir=Right  shift_bits=shift(2)  en=off  latency=0  precision=User Defined  arith_type="Signed  (2's comp)"  n_bits=bw(2)  bin_pt=b_frac(2)  quantization="Round  (unbiased: +/- Inf)"  overflow=Saturate  dbl_ovrd=off  block_type=shift
  Shift3 : xbsIndex_r4/Shift  shift_dir=Right  shift_bits=shift(3)  en=off  latency=0  precision=User Defined  arith_type="Signed  (2's comp)"  n_bits=bw(3)  bin_pt=b_frac(3)  quantization="Round  (unbiased: +/- Inf)"  overflow=Saturate  dbl_ovrd=off  block_type=shift
  Shift4 : xbsIndex_r4/Shift  shift_dir=Right  shift_bits=shift(5)  en=off  latency=0  precision=User Defined  arith_type="Signed  (2's comp)"  n_bits=bw(5)  bin_pt=b_frac(5)  quantization="Round  (unbiased: +/- Inf)"  overflow=Saturate  dbl_ovrd=off  block_type=shift
  Shift5 : xbsIndex_r4/Shift  shift_dir=Right  shift_bits=shift(6)  en=off  latency=0  precision=User Defined  arith_type="Signed  (2's comp)"  n_bits=bw(6)  bin_pt=b_frac(6)  quantization="Round  (unbiased: +/- Inf)"  overflow=Saturate  dbl_ovrd=off  block_type=shift
  Shift6 : xbsIndex_r4/Shift  shift_dir=Right  shift_bits=shift(7)  en=off  latency=0  precision=User Defined  arith_type="Signed  (2's comp)"  n_bits=bw(7)  bin_pt=b_frac(7)  quantization="Round  (unbiased: +/- Inf)"  overflow=Saturate  dbl_ovrd=off  block_type=shift
  Shift7 : xbsIndex_r4/Shift  shift_dir=Right  shift_bits=shift(8)  en=off  latency=0  precision=User Defined  arith_type="Signed  (2's comp)"  n_bits=bw(8)  bin_pt=b_frac(8)  quantization="Round  (unbiased: +/- Inf)"  overflow=Saturate  dbl_ovrd=off  block_type=shift
  Out1 : Outport
  wires:
  Constant1/1 -> Mux/3
  Constant/1 -> Mux/2
  AddSub2/1 -> AddSub1/1
  Constant2/1 -> Mux1/2
  Mux2/1 -> AddSub3/2
  Register/1 -> Shift1/1, AddSub1/2
  Shift2/1 -> AddSub2/2
  Constant5/1 -> Mux2/3
  AddSub3/1 -> AddSub2/1
  Constant4/1 -> Mux2/2
  Mux1/1 -> AddSub3/1
  AddSub1/1 -> Register/1
  Constant3/1 -> Mux1/3
  Mux/1 -> AddSub5/1
  Shift1/1 -> AddSub5/2
  AddSub5/1 -> Discrete Sigma Delta/1(In)
  AddSub4/1 -> Register1/1
  Register1/1 -> Shift/1, AddSub4/2
  Constant12/1 -> Mux6/2
  Constant10/1 -> Mux5/2
  Constant11/1 -> Mux5/3
  Register2/1 -> Shift2/1, AddSub7/2
  AddSub7/1 -> Register2/1
  Mux6/1 -> AddSub9/2
  Shift3/1 -> AddSub8/2
  Mux5/1 -> AddSub9/1
  AddSub9/1 -> AddSub8/1
  Constant13/1 -> Mux6/3
  AddSub8/1 -> AddSub7/1
  Constant16/1 -> Mux8/2
  Constant14/1 -> Mux7/2
  Constant15/1 -> Mux7/3
  Register3/1 -> Shift3/1, AddSub10/2
  AddSub10/1 -> Register3/1
  Mux8/1 -> AddSub12/2
  Shift/1 -> AddSub11/2
  Mux7/1 -> AddSub12/1
  AddSub12/1 -> AddSub11/1
  Constant17/1 -> Mux8/3
  AddSub11/1 -> AddSub10/1
  Constant7/1 -> Mux3/3
  Mux4/1 -> AddSub6/2
  Mux3/1 -> AddSub6/1
  Constant8/1 -> Mux4/2
  feedforward/1 -> Mux3/1, Mux15/1, Mux13/1, Mux11/1, Mux9/1, Mux7/1, Mux5/1, Mux/1, Mux1/1
  Constant6/1 -> Mux3/2
  Discrete Sigma Delta/1(bitstream) -> Out1/1, Mux2/1, Mux4/1, Mux16/1, Mux14/1, Mux12/1, Mux10/1, Mux8/1, Mux6/1
  Constant9/1 -> Mux4/3
  Constant18/1 -> Mux9/2
  Mux9/1 -> AddSub14/1
  Constant20/1 -> Mux10/2
  Mux10/1 -> AddSub14/2
  AddSub15/1 -> Register4/1
  Register4/1 -> Shift4/1, AddSub15/2
  Shift4/1 -> AddSub13/2
  Constant19/1 -> Mux9/3
  Constant21/1 -> Mux10/3
  AddSub13/1 -> AddSub4/1
  AddSub14/1 -> AddSub13/1
  Constant22/1 -> Mux11/2
  Mux11/1 -> AddSub17/1
  Constant24/1 -> Mux12/2
  Mux12/1 -> AddSub17/2
  AddSub18/1 -> Register5/1
  Register5/1 -> Shift5/1, AddSub18/2
  Shift5/1 -> AddSub16/2
  Constant23/1 -> Mux11/3
  Constant25/1 -> Mux12/3
  AddSub16/1 -> AddSub15/1
  AddSub17/1 -> AddSub16/1
  Constant26/1 -> Mux13/2
  Mux13/1 -> AddSub20/1
  Constant28/1 -> Mux14/2
  Mux14/1 -> AddSub20/2
  AddSub21/1 -> Register6/1
  Register6/1 -> Shift6/1, AddSub21/2
  Shift6/1 -> AddSub19/2
  Constant27/1 -> Mux13/3
  Constant29/1 -> Mux14/3
  AddSub19/1 -> AddSub18/1
  AddSub20/1 -> AddSub19/1
  Constant30/1 -> Mux15/2
  Mux15/1 -> AddSub23/1
  Constant32/1 -> Mux16/2
  Mux16/1 -> AddSub23/2
  AddSub24/1 -> Register7/1
  Register7/1 -> Shift7/1, AddSub24/2
  Shift7/1 -> AddSub22/2
  Constant31/1 -> Mux15/3
  Constant33/1 -> Mux16/3
  AddSub22/1 -> AddSub21/1
  AddSub23/1 -> AddSub22/1
  AddSub6/1 -> AddSub24/1

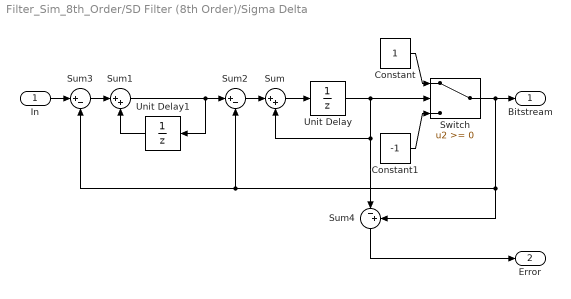
== system Filter_Sim_8th_Order/SD Filter (8th Order)/Sigma Delta ==
  In : Inport
  Constant : Constant
  Constant1 : Constant  Value=-1
  Sum : Sum  Inputs=|++
  Sum1 : Sum  Inputs=|++
  Sum2 : Sum  Inputs=|+-
  Sum3 : Sum  Inputs=|+-
  Sum4 : Sum  Inputs=|-+
  Switch : Switch
  Unit Delay : UnitDelay  SampleTime=ts
  Unit Delay1 : UnitDelay  SampleTime=ts
  Bitstream : Outport
  Error : Outport  Port=2
  wires:
  Sum4/1 -> Error/1
  Sum3/1 -> Sum1/1
  Switch/1 -> Sum4/2, Sum2/2, Sum3/2, Bitstream/1
  Constant1/1 -> Switch/3
  Unit Delay1/1 -> Sum1/2
  Sum/1 -> Unit Delay/1
  Unit Delay/1 -> Sum4/1, Sum/2, Switch/2
  Constant/1 -> Switch/1
  In/1 -> Sum3/1
  Sum2/1 -> Sum/1
  Sum1/1 -> Sum2/1, Unit Delay1/1

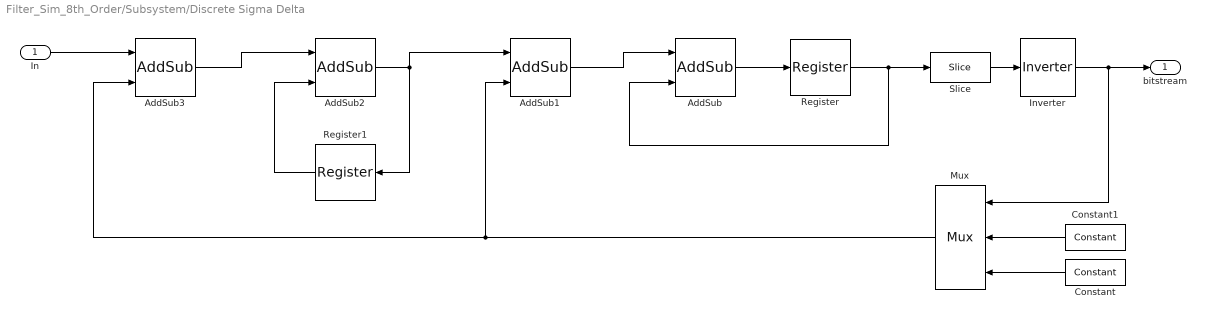
== system Filter_Sim_8th_Order/Subsystem/Discrete Sigma Delta ==
  In : Inport
  AddSub : xbsIndex_r4/AddSub  mode=Addition  use_carryin=off  use_carryout=off  en=off  latency=0  precision=User Defined  arith_type="Signed  (2's comp)"  n_bits=bw+2  bin_pt=frac  quantization="Round  (unbiased: +/- Inf)"  overflow=Saturate  use_behavioral_HDL=off  hw_selection=Fabric  pipelined=off  dbl_ovrd=off  block_type=addsub
  AddSub1 : xbsIndex_r4/AddSub  mode=Subtraction  use_carryin=off  use_carryout=off  en=off  latency=0  precision=User Defined  arith_type="Signed  (2's comp)"  n_bits=bw+2  bin_pt=frac  quantization="Round  (unbiased: +/- Inf)"  overflow=Saturate  use_behavioral_HDL=off  hw_selection=Fabric  pipelined=off  dbl_ovrd=off  block_type=addsub
  AddSub2 : xbsIndex_r4/AddSub  mode=Addition  use_carryin=off  use_carryout=off  en=off  latency=0  precision=User Defined  arith_type="Signed  (2's comp)"  n_bits=bw+2  bin_pt=frac  quantization="Round  (unbiased: +/- Inf)"  overflow=Saturate  use_behavioral_HDL=off  hw_selection=Fabric  pipelined=off  dbl_ovrd=off  block_type=addsub
  AddSub3 : xbsIndex_r4/AddSub  mode=Subtraction  use_carryin=off  use_carryout=off  en=off  latency=0  precision=User Defined  arith_type="Signed  (2's comp)"  n_bits=bw+1  bin_pt=frac  quantization="Round  (unbiased: +/- Inf)"  overflow=Saturate  use_behavioral_HDL=off  hw_selection=Fabric  pipelined=off  dbl_ovrd=off  block_type=addsub
  Constant : xbsIndex_r4/Constant  const=1.0  gui_display_data_type=Fixed-point  arith_type=Signed (2's comp)  n_bits=bw  bin_pt=frac  preci_type=Single  exp_width=8  frac_width=24  explicit_period=off  period=1  equ=P=C  opselect=C  inp2=PCIN>>17  opr=+  inp1=P  carry=CIN  dbl_ovrd=off  block_type=constant
  Constant1 : xbsIndex_r4/Constant  const=-1.0  gui_display_data_type=Fixed-point  arith_type=Signed (2's comp)  n_bits=bw  bin_pt=frac  preci_type=Single  exp_width=8  frac_width=24  explicit_period=off  period=1  equ=P=C  opselect=C  inp2=PCIN>>17  opr=+  inp1=P  carry=CIN  dbl_ovrd=off  block_type=constant
  Inverter : xbsIndex_r4/Inverter  en=off  latency=0  dbl_ovrd=off  block_type=inv
  Mux : xbsIndex_r4/Mux  inputs=2  en=off  latency=0  precision=User Defined  arith_type="Signed  (2's comp)"  n_bits=bw  bin_pt=frac  quantization="Round  (unbiased: +/- Inf)"  overflow=Saturate  dbl_ovrd=off  block_type=mux
  Register : xbsIndex_r4/Register  init=0  rst=off  en=off  dbl_ovrd=off  block_type=register
  Register1 : xbsIndex_r4/Register  init=0  rst=off  en=off  dbl_ovrd=off  block_type=register
  Slice : xbsIndex_r4/Slice  nbits=1  boolean_output=off  mode=Upper Bit Location + Width  bit1=0  base1=MSB of Input  bit0=0  base0=MSB of Input  dbl_ovrd=off  block_type=slice
  bitstream : Outport
  wires:
  AddSub1/1 -> AddSub/1
  Mux/1 -> AddSub3/2, AddSub1/2
  Inverter/1 -> Mux/1, bitstream/1
  Constant/1 -> Mux/3
  AddSub2/1 -> Register1/1, AddSub1/1
  Register1/1 -> AddSub2/2
  Constant1/1 -> Mux/2
  In/1 -> AddSub3/1
  Register/1 -> AddSub/2, Slice/1
  AddSub3/1 -> AddSub2/1
  AddSub/1 -> Register/1
  Slice/1 -> Inverter/1
